simulink model "CircuitoRLC"  (R2020a)
settings: Solver=VariableStepAuto  StartTime=0.0  StopTime=10.0  RelTol=1e-3
values from neighbouring files (symbols this model uses):
  C = 0.015    [ModeloUnicompartimental_parameters.m]    (also in RLC_parameters.m = 1)
  L = 1    [RLC_parameters.m]
  R = 20    [ModeloUnicompartimental_parameters.m]    (also in RLC_parameters.m = 2)
  V = 5    [RLC_parameters.m]
settings Model: Creator=anthony  LastModifiedBy=anthony

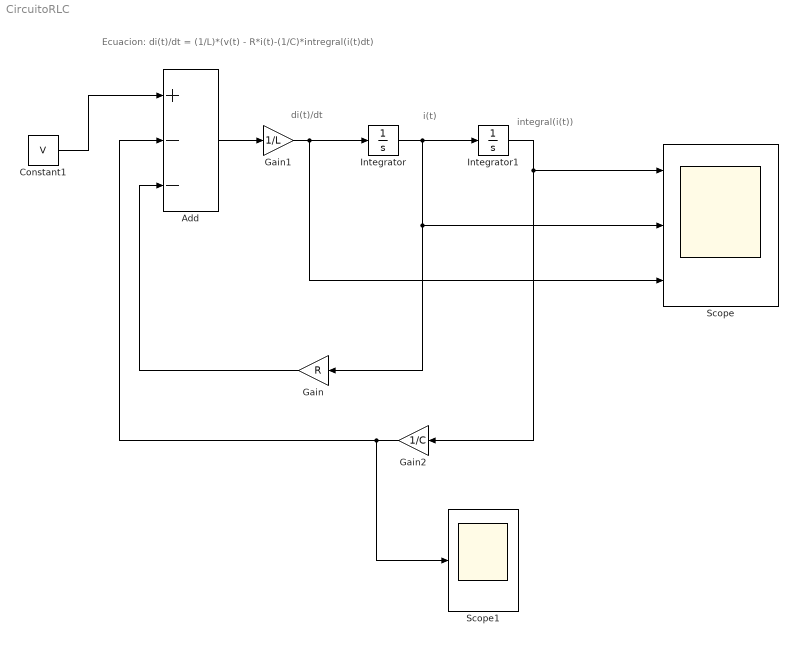
== system CircuitoRLC ==
  note: integral(i(t))
  note: i(t)
  note: di(t)/dt
  note: Ecuacion: di(t)/dt = (1/L)*(v(t) - R*i(t)-(1/C)*intregral(i(t)dt)
  Add : Sum  Inputs=+--
  Constant1 : Constant  Value=V
  Gain : Gain  Gain=R
  Gain1 : Gain  Gain=1/L
  Gain2 : Gain  Gain=1/C
  Integrator : Integrator
  Integrator1 : Integrator
  Scope : Scope  NumInputPorts=3
  Scope1 : Scope
  wires:
  Constant1/1 -> Add/1
  Gain1/1 -> Scope/3, Integrator/1
  Integrator/1 -> Integrator1/1, Scope/2, Gain/1
  Gain/1 -> Add/3
  Gain2/1 -> Scope1/1, Add/2
  Add/1 -> Gain1/1
  Integrator1/1 -> Gain2/1, Scope/1
